simulink model "RflyUdpUltraSimpleEight_Dist"  (R2022a)
settings: Solver=FixedStepDiscrete  StartTime=0.0  StopTime=inf  FixedStep=1/30  RelTol=1e-3  EnableMultiTasking=on
PreLoadFcn:
  | filepath  = fileparts(get_param(bdroot, 'FileName'))
  | cd(filepath);
undefined symbols (not defined in the file): Busy, Wait
libraries: aerolibanimutils x1
(part 2 of 2)

== matlab function RflyUdpUltraSimpleEight_Dist/Commander3 ==
  data: t input; inCMDs input; outCMDs output
function outCMDs  = fcn(t,inCMDs)

outCMDs=[-1;0;0;0;0]; % 默认空指令，不会发出

persistent mode;

if isempty(mode)
    mode=0;
end


% 进入1阶段，发送起飞指令
if mode==0 && t>1
    flag=11; % 这里对应本地起飞指令
    posX = 200; % x坐标
    posY=0; % y坐标
    posZ=-100;% z坐标
    outCMDs=[flag;posX;posY;posZ;0];
    mode=1;
end

% 10秒后，进入2模式
if mode==1 && t>5
    mode=2;
end


if mode==2
    outCMDs=inCMDs;
end

== matlab function RflyUdpUltraSimpleEight_Dist/Commander4 ==
  data: t input; inCMDs input; outCMDs output
function outCMDs  = fcn(t,inCMDs)

outCMDs=[-1;0;0;0;0]; % 默认空指令，不会发出

persistent mode;

if isempty(mode)
    mode=0;
end


% 进入1阶段，发送起飞指令
if mode==0 && t>1
    flag=11; % 这里对应本地起飞指令
    posX = 200; % x坐标
    posY=0; % y坐标
    posZ=-100;% z坐标
    outCMDs=[flag;posX;posY;posZ;0];
    mode=1;
end

% 10秒后，进入2模式
if mode==1 && t>5
    mode=2;
end


if mode==2
    outCMDs=inCMDs;
end

== matlab function RflyUdpUltraSimpleEight_Dist/Commander5 ==
  data: t input; inCMDs input; outCMDs output
function outCMDs  = fcn(t,inCMDs)

outCMDs=[-1;0;0;0;0]; % 默认空指令，不会发出

persistent mode;

if isempty(mode)
    mode=0;
end


% 进入1阶段，发送起飞指令
if mode==0 && t>1
    flag=11; % 这里对应本地起飞指令
    posX = 200; % x坐标
    posY=0; % y坐标
    posZ=-100;% z坐标
    outCMDs=[flag;posX;posY;posZ;0];
    mode=1;
end

% 10秒后，进入2模式
if mode==1 && t>5
    mode=2;
end


if mode==2
    outCMDs=inCMDs;
end

== matlab function RflyUdpUltraSimpleEight_Dist/Commander6 ==
  data: t input; inCMDs input; outCMDs output
function outCMDs  = fcn(t,inCMDs)

outCMDs=[-1;0;0;0;0]; % 默认空指令，不会发出

persistent mode;

if isempty(mode)
    mode=0;
end


% 进入1阶段，发送起飞指令
if mode==0 && t>1
    flag=11; % 这里对应本地起飞指令
    posX = 200; % x坐标
    posY=0; % y坐标
    posZ=-100;% z坐标
    outCMDs=[flag;posX;posY;posZ;0];
    mode=1;
end

% 10秒后，进入2模式
if mode==1 && t>5
    mode=2;
end


if mode==2
    outCMDs=inCMDs;
end

== matlab function RflyUdpUltraSimpleEight_Dist/Commander7 ==
  data: t input; inCMDs input; outCMDs output
function outCMDs  = fcn(t,inCMDs)

outCMDs=[-1;0;0;0;0]; % 默认空指令，不会发出

persistent mode;

if isempty(mode)
    mode=0;
end


% 进入1阶段，发送起飞指令
if mode==0 && t>1
    flag=11; % 这里对应本地起飞指令
    posX = 200; % x坐标
    posY=0; % y坐标
    posZ=-100;% z坐标
    outCMDs=[flag;posX;posY;posZ;0];
    mode=1;
end

% 10秒后，进入2模式
if mode==1 && t>5
    mode=2;
end


if mode==2
    outCMDs=inCMDs;
end

== matlab function RflyUdpUltraSimpleEight_Dist/Commander8 ==
  data: t input; inCMDs input; outCMDs output
function outCMDs  = fcn(t,inCMDs)

outCMDs=[-1;0;0;0;0]; % 默认空指令，不会发出

persistent mode;

if isempty(mode)
    mode=0;
end


% 进入1阶段，发送起飞指令
if mode==0 && t>1
    flag=11; % 这里对应本地起飞指令
    posX = 200; % x坐标
    posY=0; % y坐标
    posZ=-100;% z坐标
    outCMDs=[flag;posX;posY;posZ;0];
    mode=1;
end

% 10秒后，进入2模式
if mode==1 && t>5
    mode=2;
end


if mode==2
    outCMDs=inCMDs;
end

== matlab function RflyUdpUltraSimpleEight_Dist/Commander9 ==
  data: t input; inCMDs input; outCMDs output
function outCMDs  = fcn(t,inCMDs)

outCMDs=[-1;0;0;0;0]; % 默认空指令，不会发出

persistent mode;

if isempty(mode)
    mode=0;
end


% 进入1阶段，发送起飞指令
if mode==0 && t>1
    flag=11; % 这里对应本地起飞指令
    posX = 200; % x坐标
    posY=0; % y坐标
    posZ=-100;% z坐标
    outCMDs=[flag;posX;posY;posZ;0];
    mode=1;
end

% 10秒后，进入2模式
if mode==1 && t>5
    mode=2;
end


if mode==2
    outCMDs=inCMDs;
end

== matlab function RflyUdpUltraSimpleEight_Dist/Commander10 ==
  data: t input; inCMDs input; outCMDs output
function outCMDs  = fcn(t,inCMDs)

outCMDs=[-1;0;0;0;0]; % 默认空指令，不会发出

persistent mode;

if isempty(mode)
    mode=0;
end


% 进入1阶段，发送起飞指令
if mode==0 && t>1
    flag=11; % 这里对应本地起飞指令
    posX = 200; % x坐标
    posY=0; % y坐标
    posZ=-100;% z坐标
    outCMDs=[flag;posX;posY;posZ;0];
    mode=1;
end

% 10秒后，进入2模式
if mode==1 && t>5
    mode=2;
end


if mode==2
    outCMDs=inCMDs;
end
